simulink model "Abstract_Transmission"  (R2014b)
settings: Solver=ode45  StartTime=0.0  StopTime=10.0  RelTol=1e-3
undefined symbols (not defined in the file): DCT_Param
libraries: fl_lib x6, sdl_lib x2, nesl_utility x2
Description:
  | Copyright 2014 The MathWorks, Inc.
settings Model: Creator=smiller  LastModifiedBy=psanghvi
settings DataIOCC: SignalLoggingSaveFormat=ModelDataLogs
settings OptimizationCC: ExpressionDepthLimit=2147483647
settings DebuggingCC: UnderspecifiedInitializationDetection=Classic  MergeDetectMultiDrivingBlocksExec=none  FcnCallInpInsideContextMsg=UseLocalSettings  StateNameClashWarn=warning
settings GRTTargetCC: CombineOutputUpdateFcns=off  GRTInterface=on

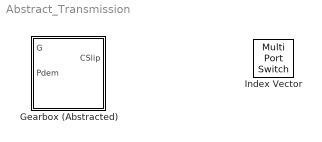
== system Abstract_Transmission ==
  Gearbox (Abstracted) : Subsystem
  Index Vector : MultiPortSwitch  DataPortOrder=Zero-based contiguous  Inputs=1  zeroidx=on

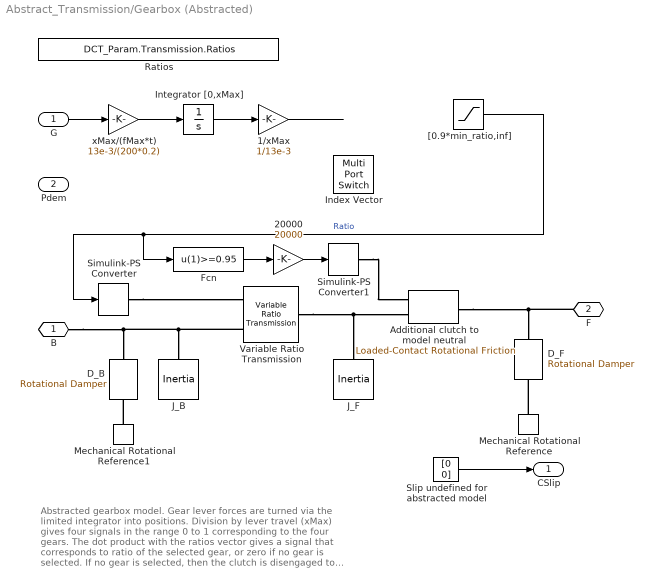
== system Abstract_Transmission/Gearbox (Abstracted) ==
  note: Abstracted gearbox model. Gear lever forces are turned
      | via the limited integrator into positions. Division
      | by lever travel (xMax) gives four signals in the range
      | 0 to 1 corresponding to the four gears. The dot
      | product with the ratios vector gives a signal that
      | corresponds to ratio of the selected gear, or zero if
      | no gear is selected. If no gear is selected, then the
      | clutch is disengaged to represent neutral.
  G : Inport
  Pdem : Inport  Port=2
  1/xMax : Gain  Gain=1/13e-3  SaturateOnIntegerOverflow=on  OutDataTypeStr=Inherit: Same as input  ParamDataTypeStr=Inherit: Same as input
  20000 : Gain  Gain=20000  SaturateOnIntegerOverflow=on  OutDataTypeStr=Inherit: Same as input  ParamDataTypeStr=Inherit: Same as input
  Additional clutch to model neutral : sdl_lib/Brakes & Detents/Rotational/Loaded-Contact Rotational Friction  geometry_model=1  r_eff=300 mm  d_o=150 mm  d_i=100 mm  friction_model=1  mu_coulomb=0.46  mu_w_vector=[ 0 0.1 0.2 0.3 0.4 0.5 1 2 5 10 100 1000 ] rad/s  mu_coulomb_vector=[ 0.29 0.28 0.26 0.22 0.21 0.2 0.2 0.19 0.19 0.19 0.19 0.19 ]  mu_interp_method=1  mu_extrap_method=1  mu_static=0.5  w_tol=0.001 rad/s  force_min=100 N  mu_visc=0 N*m/(rad/s)  initial_state_locked=0
  D_B : fl_lib/Mechanical/Rotational Elements/Rotational Damper  D=0.01 N*m/(rad/s)  w_specify=off  w_priority=High  w=0 rad/s  t_specify=off  t_priority=High  t=0 N*m
  D_F : fl_lib/Mechanical/Rotational Elements/Rotational Damper  D=0.01 N*m/(rad/s)  w_specify=off  w_priority=High  w=0 rad/s  t_specify=off  t_priority=High  t=0 N*m
  Fcn : Fcn  Expr=u(1)>=0.95
  Index Vector : MultiPortSwitch  DataPortOrder=Zero-based contiguous  Inputs=1  zeroidx=on
  Integrator [0,xMax] : Integrator  LimitOutput=on  UpperSaturationLimit=13e-3  LowerSaturationLimit=0
  J_B : fl_lib/Mechanical/Rotational Elements/Inertia  inertia=0.026 kg*m^2  w_specify=on  w_priority=High  w=0 rad/s  t_specify=off  t_priority=High  t=0 N*m
  J_F : fl_lib/Mechanical/Rotational Elements/Inertia  inertia=0.034 kg*m^2  w_specify=on  w_priority=High  w=0 rad/s  t_specify=off  t_priority=High  t=0 N*m
  Mechanical Rotational Reference : fl_lib/Mechanical/Rotational Elements/Mechanical Rotational Reference
  Mechanical Rotational Reference1 : fl_lib/Mechanical/Rotational Elements/Mechanical Rotational Reference
  Ratios : Constant  Value=DCT_Param.Transmission.Ratios  VectorParams1D=off
  Simulink-PS Converter : nesl_utility/Simulink-PS Converter  PhysicalDomain=network_engine_domain  SubClassName=ps_input  LeftPortType=input  RightPortType=output  PseudoPeriodic=off  Frequencies=[]  NoiseDistribution=none  NoiseParameters=[]  Unit=1  AffineConversion=off  InputFiltering=off  SimscapeFilterOrder=1  InputFilterTimeConstant=.001  UdotUserProvided=0
  Simulink-PS Converter1 : nesl_utility/Simulink-PS Converter  PhysicalDomain=network_engine_domain  SubClassName=ps_input  LeftPortType=input  RightPortType=output  PseudoPeriodic=off  Frequencies=[]  NoiseDistribution=none  NoiseParameters=[]  Unit=1  AffineConversion=off  InputFiltering=off  SimscapeFilterOrder=1  InputFilterTimeConstant=.001  UdotUserProvided=0
  Slip undefined for abstracted model : Constant  Value=[0 0]
  Variable Ratio Transmission : sdl_lib/Couplings & Drives/Variable Ratio Transmission  rotation_direction=1  kp=1e+5 N*m/rad  kv=10 N*m/(rad/s)  initial_torque=0 N*m  losses_model=1  efficiency=0.85  mu_visc=[ 0 0 ] N*m/(rad/s)  w_thr=0.01 rad/s
  "[0.9*min_ratio,inf]" : Saturate  UpperLimit=inf  LowerLimit=0.9
  xMax/(fMax*t) : Gain  Gain=13e-3/(200*0.2)  SaturateOnIntegerOverflow=on  OutDataTypeStr=Inherit: Same as input  ParamDataTypeStr=Inherit: Same as input
  B : PMIOPort  Port=1  Side=Left
  F : PMIOPort  Port=2  Side=Right
  CSlip : Outport
  wires:
  20000/1 -> Simulink-PS Converter1/1
  Fcn/1 -> 20000/1
  "[0.9*min_ratio,inf]"/1 -> Fcn/1, Simulink-PS Converter/1  "Ratio"
  G/1 -> xMax/(fMax*t)/1
  xMax/(fMax*t)/1 -> Integrator [0,xMax]/1
  Integrator [0,xMax]/1 -> 1/xMax/1
  1/xMax/1 -> ?
  ? -> "[0.9*min_ratio,inf]"/1
  Slip undefined for abstracted model/1 -> CSlip/1
  connections:
  Simulink-PS Converter1/RConn1 -- Additional clutch to model neutral/LConn1
  Variable Ratio Transmission/RConn1 -- Additional clutch to model neutral/LConn2 -- J_F/LConn1
  Simulink-PS Converter/RConn1 -- Variable Ratio Transmission/LConn1
  Variable Ratio Transmission/LConn2 -- B/RConn1 -- D_B/LConn1 -- J_B/LConn1
  Mechanical Rotational Reference/LConn1 -- D_F/RConn1
  Mechanical Rotational Reference1/LConn1 -- D_B/RConn1
  Additional clutch to model neutral/RConn1 -- D_F/LConn1 -- F/RConn1
